simulink model "part1"  (R2020b)
settings: Solver=VariableStepAuto  StartTime=0.0  StopTime=2  RelTol=1e-3
libraries: simulink_extras x4
settings Model: Creator=Catherina Liu  LastModifiedBy=28217

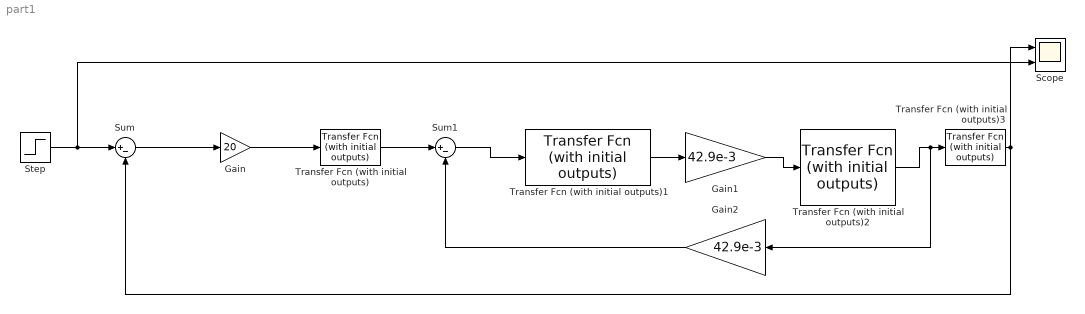
== system part1 ==
  Gain : Gain  Gain=20
  Gain1 : Gain  Gain=42.9e-3
  Gain2 : Gain  Gain=42.9e-3
  Scope : Scope  NumInputPorts=2
  Step : Step  After=pi/2  SampleTime=0
  Sum : Sum  Inputs=|+-
  Sum1 : Sum  Inputs=|+-
  Transfer Fcn (with initial outputs) : simulink_extras/Additional Linear/Transfer Fcn (with initial outputs)  N=[5000]  D="[1  5000]"  Y0=.5  U0=0
  Transfer Fcn (with initial outputs)1 : simulink_extras/Additional Linear/Transfer Fcn (with initial outputs)  N=[1]  D="[0.514e-3  2.68]"  Y0=.5  U0=0
  Transfer Fcn (with initial outputs)2 : simulink_extras/Additional Linear/Transfer Fcn (with initial outputs)  N=[1]  D=[21.2e-7 7e-4]  Y0=.5  U0=0
  Transfer Fcn (with initial outputs)3 : simulink_extras/Additional Linear/Transfer Fcn (with initial outputs)  N=[1]  D="[1  0]"  Y0=.5  U0=0
  wires:
  Gain/1 -> Transfer Fcn (with initial outputs)/1
  Transfer Fcn (with initial outputs)/1 -> Sum1/1
  Sum1/1 -> Transfer Fcn (with initial outputs)1/1
  Transfer Fcn (with initial outputs)1/1 -> Gain1/1
  Gain1/1 -> Transfer Fcn (with initial outputs)2/1
  Gain2/1 -> Sum1/2
  Transfer Fcn (with initial outputs)2/1 -> Gain2/1, Transfer Fcn (with initial outputs)3/1
  Transfer Fcn (with initial outputs)3/1 -> Sum/2, Scope/1
  Sum/1 -> Gain/1
  Step/1 -> Scope/2, Sum/1
